simulink subsystem "PieroControladoV"  (R2023b)
settings: Solver=VariableStepAuto  StartTime=0.0  StopTime=10.0  RelTol=1e-3
settings Model: Creator=Usuario_UMA  LastModifiedBy=Manuel

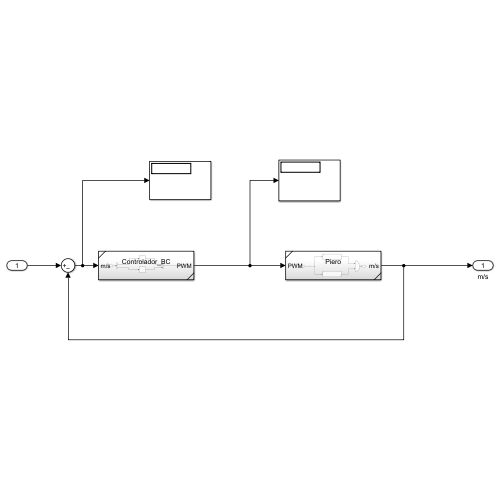
[thumbnail: Simulink's stored preview of the top-level diagram]
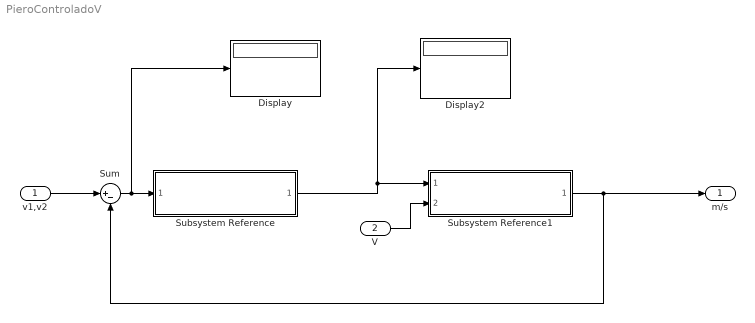
== system PieroControladoV ==
  v1,v2 : Inport
  V : Inport  Port=2
  Display : Display
  Display2 : Display
  Subsystem Reference : Subsystem  ReferencedSubsystem=Controlador_BC
  Subsystem Reference1 : Subsystem  ReferencedSubsystem=Piero
  Sum : Sum  Inputs=|+-
  m/s : Outport
  wires:
  Sum/1 -> Display/1, Subsystem Reference/1
  v1,v2/1 -> Sum/1
  Subsystem Reference/1 -> Display2/1, Subsystem Reference1/1
  Subsystem Reference1/1 -> m/s/1, Sum/2
  V/1 -> Subsystem Reference1/2
